simulink model "sampleModel1673"  (R2023a)
settings: Solver=VariableStepAuto  StartTime=0.0  StopTime=10.0  RelTol=1e-3
libraries: hdlsllib x6, simulink x5
settings Model: Creator=user1  LastModifiedBy=user1

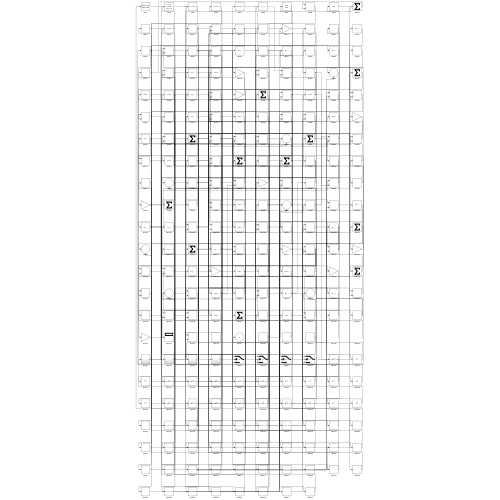
[thumbnail: Simulink's stored preview of the top-level diagram]
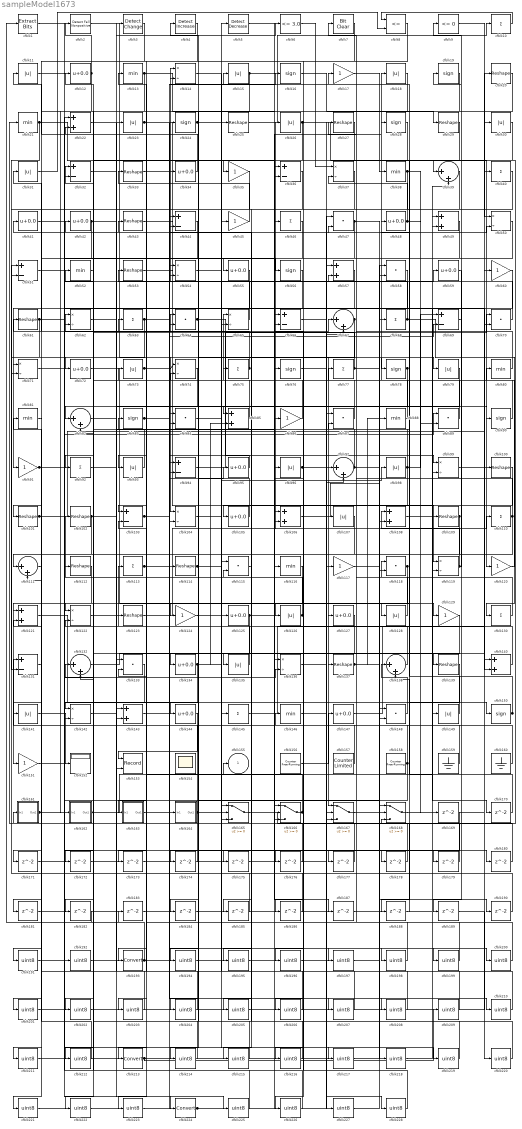
== system sampleModel1673 ==
  cfblk1 : simulink/Logic and Bit Operations/Extract Bits  bitsToExtract=Upper half  numBits=8  bitIdxRange=[0 7]  outScalingMode=Preserve fixed-point scaling
      settings: LibrarySourceBlock=|
      | hdlsllib/Logic and Bit
      | Operations/Extract Bits
  cfblk{10,40,46,63,68,75,77,92,110,113,130,145} (12 alike) : Sum  Inputs=+
  cfblk{20,25,27,29,33,43,53,61,100..102,109,112,114,123,137,139} (17 alike) : Reshape
  cfblk{32,36,44,51,66,69,94,103,131} (9 alike) : Sum  Inputs=+-
  cfblk{14,37,50,54,62,65,71,74,99,104,119,122,136,142} (14 alike) : Product  Inputs=*/  RndMeth=Zero  SaturateOnIntegerOverflow=on
  cfblk{12,34,41..42,48,55,59,72,95,105,125,127,134,144,147} (15 alike) : Bias  Bias=0.0  SaturateOnIntegerOverflow=off
  cfblk{22,49,57,85,106,108,121,140,143} (9 alike) : Sum
  cfblk{11,15,18,23,26,30..31,73,79,93,96,98,107,126,128,135,141,149} (18 alike) : Abs  SaturateOnIntegerOverflow=off
  cfblk{39,67,82,97,111,132,138} (7 alike) : Sum  Inputs=|++
  cfblk{47,58,64,70,84,87,89,115,118,133,148} (11 alike) : DotProduct  OutDataTypeStr=Inherit: Inherit via internal rule
  cfblk{13,21,38,52,80..81,88,116,146} (9 alike) : MinMax
  cfblk{17,35,45,60,86,91,117,120,124,129,151} (11 alike) : Gain
  cfblk{16,19,24,28,56,76,78,83,90,150} (10 alike) : Signum
  cfblk152 : Display
  cfblk153 : Record  FileSettingsInternal="{\"entries\":[{\"content\":{\"excelSettings\":{\"content\":{},\"type\":\"Streamout.ExcelSettings\"}},\"type\":\"Streamout.FileSettingStorage\",\"uuid\":\"\"}],\"packageUris\":[\"http:\\/\\/schema.mathworks.com\\/mf0\\/streamout_blocks\\/R2020a\"],\"version\":\"1.0\"}"  Layout=[1 1]  SignalsInternal="{\"entries\":[{\"content\":{\"signals\":[{\"content\":{\"blockPath\":[],\"dimensions\":[1],\"domain\":\"\",\"lineColor\":\"#a2142f\",\"plots\":[1],\"port\":1,\"signalID\":2764,\"signalName\":\"XY Graph:1\"},\"type\":\"RecordBlkView.Signal\",\"uuid\":\"\"},{\"content\":{\"blockPath\":[],\"dimensions\":[1],\"domain\":\"\",\"lineColor\":\"#139fff\",\"plots\":[1],\"port\":2,\"signalID\":2767,\"signalName\":\"XY Graph:2\"},\"type\":\"RecordBlkView.Signal\",\"uuid\":\"\"}]},\"type\":\"RecordBlkView.InputSignals\",\"uuid\":\"\"}],\"packageUris\":[\"http:\\/\\/schema.mathworks.com\\/mf0\\/streamout_blocks\\/R2020a\"],\"version\":\"1.0\"}"  VisualizationBindings="{\"xyplotplugin\":{\"info\":[{\"series\":[{\"bindingParametersList\":[{\"parameter\":\"X-Axis\",\"signalID\":2764,\"signalName\":\"XY Graph:1\"},{\"parameter\":\"Y-Axis\",\"signalID\":2767,\"signalName\":\"XY Graph:2\"}],\"seriesID\":48167}],\"subplotID\":1}]}}"  CompatibilityTag=XY  st=-1
  cfblk154 : Scope
      settings: Floating=on
  cfblk156 : hdlsllib/Sources/Counter Free-Running  NumBits=16  tsamp=-1
  cfblk157 : hdlsllib/Sources/Counter Limited  uplimit=7  tsamp=-1
  cfblk158 : hdlsllib/Sources/Counter Free-Running  NumBits=16  tsamp=-1
  cfblk159 : Ground
  cfblk160 : Ground
  cfblk161 : Subsystem
      settings: LibrarySourceBlock=|
      | hdlsllib/Ports &
      | Subsystems/Subsystem
  cfblk162 : Subsystem
      settings: LibrarySourceBlock=|
      | hdlsllib/Ports &
      | Subsystems/Subsystem
  cfblk163 : Subsystem
      settings: LibrarySourceBlock=|
      | hdlsllib/Ports &
      | Subsystems/Subsystem
  cfblk164 : Subsystem
      settings: LibrarySourceBlock=|
      | hdlsllib/Ports &
      | Subsystems/Subsystem
  cfblk{165..168} (4 alike) : Switch  SaturateOnIntegerOverflow=off  InputSameDT=off
  cfblk{169..190} (22 alike) : Delay  SampleTime=1
  cfblk{191..192,194..212,214..223,225..228} (35 alike) : DataTypeConversion  OutDataTypeStr=uint8  SaturateOnIntegerOverflow=off  RndMeth=Floor
  cfblk193 : DataTypeConversion  SaturateOnIntegerOverflow=off  RndMeth=Floor
  cfblk2 : hdlsllib/Logic and Bit Operations/Detect Fall Nonpositive  vinit=0  OutDataTypeStr=boolean
  cfblk213 : DataTypeConversion  SaturateOnIntegerOverflow=off  RndMeth=Floor
  cfblk224 : DataTypeConversion  SaturateOnIntegerOverflow=off  RndMeth=Floor
  cfblk3 : simulink/Logic and Bit Operations/Detect Change  vinit=0  OutDataTypeStr=boolean
      settings: LibrarySourceBlock=|
      | hdlsllib/Logic and Bit
      | Operations/Detect
      | Change
  cfblk4 : simulink/Logic and Bit Operations/Detect Increase  vinit=0.0  OutDataTypeStr=boolean
      settings: LibrarySourceBlock=|
      | hdlsllib/Logic and Bit
      | Operations/Detect
      | Increase
  cfblk5 : simulink/Logic and Bit Operations/Detect Decrease  vinit=0.0  OutDataTypeStr=boolean
      settings: LibrarySourceBlock=|
      | hdlsllib/Logic and Bit
      | Operations/Detect
      | Decrease
  cfblk6 : hdlsllib/Logic and Bit Operations/Compare To Constant  relop=<=  const=3.0  OutDataTypeStr=boolean
  cfblk7 : simulink/Logic and Bit Operations/Bit Clear  iBit=0
      settings: LibrarySourceBlock=|
      | hdlsllib/Logic and Bit
      | Operations/Bit Clear
  cfblk8 : RelationalOperator  Operator=<=  OutDataTypeStr=boolean  InputSameDT=off
  cfblk9 : hdlsllib/Logic and Bit Operations/Compare To Zero  relop=<=  OutDataTypeStr=boolean
  cfblk155 : Outport  VectorParamsAs1DForOutWhenUnconnected=off
  wires:
  cfblk72/1 -> cfblk126/1
  cfblk98/1 -> cfblk105/1, cfblk69/1, cfblk61/1
  cfblk10/1 -> cfblk8/1
  cfblk150/1 -> cfblk113/1, cfblk14/2
  cfblk64/1 -> cfblk99/1, cfblk79/1
  cfblk86/1 -> cfblk42/1
  cfblk88/1 -> cfblk18/1
  cfblk67/1 -> cfblk167/1, cfblk134/1
  cfblk104/1 -> cfblk98/1
  cfblk75/1 -> cfblk62/1, cfblk31/1
  cfblk90/1 -> cfblk73/1
  cfblk68/1 -> cfblk130/1, cfblk54/1
  cfblk15/1 -> cfblk162/1(In1), cfblk187/1
  cfblk2/1 -> cfblk104/1
  cfblk123/1 -> cfblk5/1
  cfblk166/1 -> cfblk63/1, cfblk155/1
  cfblk165/1 -> cfblk39/1
  cfblk6/1 -> cfblk37/1
  cfblk121/1 -> cfblk150/1
  cfblk39/1 -> cfblk82/1
  cfblk124/1 -> cfblk25/1
  cfblk44/1 -> cfblk213/1
  cfblk31/1 -> cfblk8/2
  cfblk23/1 -> cfblk119/1, cfblk78/1, cfblk207/1
  cfblk128/1 -> cfblk118/1
  cfblk141/1 -> cfblk152/1
  cfblk137/1 -> cfblk88/1, cfblk190/1
  cfblk26/1 -> cfblk120/1, cfblk153/2, cfblk210/1
  cfblk55/1 -> cfblk103/1
  cfblk132/1 -> cfblk135/1
  cfblk65/1 -> cfblk14/1
  cfblk25/1 -> cfblk10/1
  cfblk100/1 -> cfblk127/1
  cfblk125/1 -> cfblk28/1, cfblk132/2
  cfblk50/1 -> cfblk124/1
  cfblk157/1 -> cfblk64/1
  cfblk14/1 -> cfblk45/1
  cfblk38/1 -> cfblk131/2, cfblk169/1
  cfblk145/1 -> cfblk60/1
  cfblk60/1 -> cfblk91/1
  cfblk95/1 -> cfblk94/1
  cfblk112/1 -> cfblk151/1
  cfblk99/1 -> cfblk100/1
  cfblk164/1(Out1) -> cfblk21/1, cfblk50/2, cfblk132/1
  cfblk82/1 -> cfblk23/1
  cfblk160/1 -> cfblk27/1
  cfblk41/1 -> cfblk55/1
  cfblk73/1 -> cfblk74/1, cfblk166/3
  cfblk69/1 -> cfblk19/1
  cfblk27/1 -> cfblk94/2
  cfblk96/1 -> cfblk57/1, cfblk228/1
  cfblk102/1 -> cfblk111/1, cfblk86/1
  cfblk109/1 -> cfblk118/2, cfblk203/1
  cfblk168/1 -> cfblk20/1
  cfblk113/1 -> cfblk26/1, cfblk69/2
  cfblk43/1 -> cfblk119/2
  cfblk110/1 -> cfblk57/2, cfblk188/1, cfblk201/1
  cfblk156/1 -> cfblk147/1
  cfblk106/1 -> cfblk68/1
  cfblk63/1 -> cfblk114/1, cfblk46/1, cfblk71/2
  cfblk30/1 -> cfblk128/1
  cfblk147/1 -> cfblk99/2
  cfblk130/1 -> cfblk77/1
  cfblk89/1 -> cfblk65/1
  cfblk4/1 -> cfblk193/1
  cfblk35/1 -> cfblk104/2
  cfblk97/1 -> cfblk54/2, cfblk199/1
  cfblk52/1 -> cfblk122/1
  cfblk47/1 -> cfblk148/1, cfblk226/1
  cfblk45/1 -> cfblk13/1
  cfblk94/1 -> cfblk70/1
  cfblk61/1 -> cfblk144/1, cfblk71/1
  cfblk101/1 -> cfblk40/1, cfblk166/2, cfblk59/1
  cfblk18/1 -> cfblk72/1
  cfblk126/1 -> cfblk102/1, cfblk96/1
  cfblk24/1 -> cfblk56/1, cfblk129/1
  cfblk103/1 -> cfblk47/2, cfblk95/1
  cfblk158/1 -> cfblk131/1, cfblk204/1
  cfblk54/1 -> cfblk145/1
  cfblk80/1 -> cfblk53/1
  cfblk105/1 -> cfblk24/1
  cfblk13/1 -> cfblk136/1, cfblk111/2
  cfblk120/1 -> cfblk80/1
  cfblk70/1 -> cfblk48/1
  cfblk46/1 -> cfblk141/1
  cfblk119/1 -> cfblk108/1, cfblk9/1
  cfblk144/1 -> cfblk153/1
  cfblk159/1 -> cfblk34/1
  cfblk17/1 -> cfblk38/1
  cfblk149/1 -> cfblk87/2
  cfblk107/1 -> cfblk142/1
  cfblk16/1 -> cfblk29/1
  cfblk140/1 -> cfblk43/1
  cfblk20/1 -> cfblk93/1
  cfblk148/1 -> cfblk138/1
  cfblk34/1 -> cfblk11/1
  cfblk33/1 -> cfblk137/1
  cfblk85/1 -> cfblk32/1
  cfblk9/1 -> cfblk50/1
  cfblk91/1 -> cfblk217/1, cfblk225/1
  cfblk32/1 -> cfblk35/1
  cfblk114/1 -> cfblk110/1, cfblk177/1
  cfblk87/1 -> cfblk32/2
  cfblk22/1 -> cfblk224/1
  cfblk142/1 -> cfblk67/1
  cfblk48/1 -> cfblk7/1, cfblk89/2
  cfblk62/1 -> cfblk165/2
  cfblk77/1 -> cfblk52/1, cfblk140/2
  cfblk143/1 -> cfblk16/1
  cfblk122/1 -> cfblk143/2
  cfblk36/1 -> cfblk85/1
  cfblk83/1 -> cfblk139/1, cfblk15/1
  cfblk138/1 -> cfblk74/2
  cfblk42/1 -> cfblk121/1, cfblk90/1
  cfblk53/1 -> cfblk140/1
  cfblk135/1 -> cfblk112/1
  cfblk162/1(Out1) -> cfblk123/1, cfblk109/1
  cfblk78/1 -> cfblk106/2, cfblk142/2
  cfblk93/1 -> cfblk41/1
  cfblk12/1 -> cfblk2/1, cfblk101/1
  cfblk167/1 -> cfblk108/2
  cfblk161/1(Out1) -> cfblk64/2, cfblk89/1
  cfblk151/1 -> cfblk136/2
  cfblk92/1 -> cfblk6/1
  cfblk74/1 -> cfblk92/1
  cfblk118/1 -> cfblk163/1(In1), cfblk185/1, cfblk194/1
  cfblk21/1 -> cfblk36/2, cfblk51/2
  cfblk11/1 -> cfblk70/2
  cfblk1/1 -> cfblk168/2
  cfblk134/1 -> cfblk65/2, cfblk85/2, cfblk182/1
  cfblk108/1 -> cfblk170/1
  cfblk170/1 -> cfblk138/2
  cfblk8/1 -> cfblk171/1
  cfblk171/1 -> cfblk165/1
  cfblk56/1 -> cfblk172/1
  cfblk172/1 -> cfblk143/1
  cfblk129/1 -> cfblk173/1
  cfblk173/1 -> cfblk97/2
  cfblk19/1 -> cfblk174/1
  cfblk174/1 -> cfblk122/2
  cfblk71/1 -> cfblk175/1
  cfblk175/1 -> cfblk106/1
  cfblk40/1 -> cfblk176/1
  cfblk176/1 -> cfblk62/2
  cfblk177/1 -> cfblk82/2
  cfblk139/1 -> cfblk178/1
  cfblk178/1 -> cfblk168/1
  cfblk5/1 -> cfblk179/1
  cfblk179/1 -> cfblk37/2
  cfblk136/1 -> cfblk180/1
  cfblk180/1 -> cfblk47/1
  cfblk111/1 -> cfblk181/1
  cfblk181/1 -> cfblk165/3
  cfblk182/1 -> cfblk1/1
  cfblk183/1 -> cfblk166/1
  cfblk79/1 -> cfblk184/1
  cfblk184/1 -> cfblk39/2
  cfblk185/1 -> cfblk103/2
  cfblk28/1 -> cfblk186/1
  cfblk186/1 -> cfblk51/1
  cfblk188/1 -> cfblk168/3
  cfblk59/1 -> cfblk189/1
  cfblk190/1 -> cfblk33/1
  cfblk3/1 -> cfblk191/1
  cfblk191/1 -> cfblk125/1
  cfblk51/1 -> cfblk192/1
  cfblk192/1 -> cfblk3/1
  cfblk193/1 -> cfblk183/1, cfblk121/2, cfblk107/1
  cfblk194/1 -> cfblk4/1
  cfblk58/1 -> cfblk195/1
  cfblk195/1 -> cfblk36/1
  cfblk127/1 -> cfblk196/1
  cfblk196/1 -> cfblk58/1
  cfblk163/1(Out1) -> cfblk197/1
  cfblk197/1 -> cfblk58/2
  cfblk76/1 -> cfblk198/1
  cfblk198/1 -> cfblk17/1
  cfblk199/1 -> cfblk76/1
  cfblk117/1 -> cfblk200/1
  cfblk200/1 -> cfblk83/1
  cfblk201/1 -> cfblk117/1
  cfblk133/1 -> cfblk202/1
  cfblk202/1 -> cfblk164/1(In1)
  cfblk203/1 -> cfblk133/1
  cfblk204/1 -> cfblk133/2
  cfblk115/1 -> cfblk205/1
  cfblk205/1 -> cfblk30/1
  cfblk7/1 -> cfblk206/1
  cfblk206/1 -> cfblk115/1
  cfblk207/1 -> cfblk115/2
  cfblk66/1 -> cfblk208/1
  cfblk208/1 -> cfblk161/1(In1)
  cfblk209/1 -> cfblk66/1
  cfblk210/1 -> cfblk66/2
  cfblk81/1 -> cfblk211/1
  cfblk211/1 -> cfblk87/1
  cfblk29/1 -> cfblk212/1
  cfblk212/1 -> cfblk81/1
  cfblk213/1 -> cfblk209/1, cfblk149/1, cfblk97/1
  cfblk169/1 -> cfblk214/1
  cfblk214/1 -> cfblk44/1
  cfblk37/1 -> cfblk215/1
  cfblk215/1 -> cfblk44/2
  cfblk49/1 -> cfblk216/1
  cfblk216/1 -> cfblk12/1
  cfblk217/1 -> cfblk49/1
  cfblk187/1 -> cfblk218/1
  cfblk218/1 -> cfblk49/2
  cfblk84/1 -> cfblk219/1
  cfblk219/1 -> cfblk75/1
  cfblk189/1 -> cfblk220/1
  cfblk220/1 -> cfblk84/1
  cfblk131/1 -> cfblk221/1
  cfblk221/1 -> cfblk84/2
  cfblk116/1 -> cfblk222/1
  cfblk222/1 -> cfblk167/2
  cfblk57/1 -> cfblk223/1
  cfblk223/1 -> cfblk116/1
  cfblk224/1 -> cfblk67/2, cfblk167/3
  cfblk225/1 -> cfblk22/1
  cfblk226/1 -> cfblk22/2
  cfblk146/1 -> cfblk227/1
  cfblk227/1 -> cfblk148/2
  cfblk228/1 -> cfblk146/1

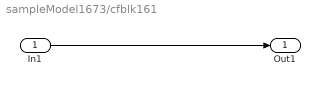
== system sampleModel1673/cfblk161 ==
  In1 : Inport
  Out1 : Outport
  wires:
  In1/1 -> Out1/1

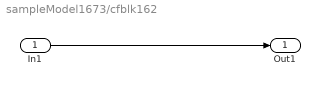
== system sampleModel1673/cfblk162 ==
  In1 : Inport
  Out1 : Outport
  wires:
  In1/1 -> Out1/1

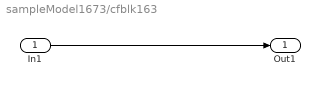
== system sampleModel1673/cfblk163 ==
  In1 : Inport
  Out1 : Outport
  wires:
  In1/1 -> Out1/1

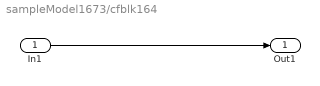
== system sampleModel1673/cfblk164 ==
  In1 : Inport
  Out1 : Outport
  wires:
  In1/1 -> Out1/1
